simulink model "truck_fra_siden"  (R2023b)
settings: Solver=VariableStepAuto  StartTime=0.0  StopTime=100  MaxStep=0.01  RelTol=1e-3
values from neighbouring files (symbols this model uses):
  K_i = 10    [truck_fra_siden_script.m]
  K_p = 1400    [truck_fra_siden_script.m]
  v_r = 20    [truck_fra_siden_script.m]
settings Model: PacingRate=2  Creator=hansae  LastModifiedBy=fredr
settings SolverCC: AlgebraicLoopSolver=TrustRegion

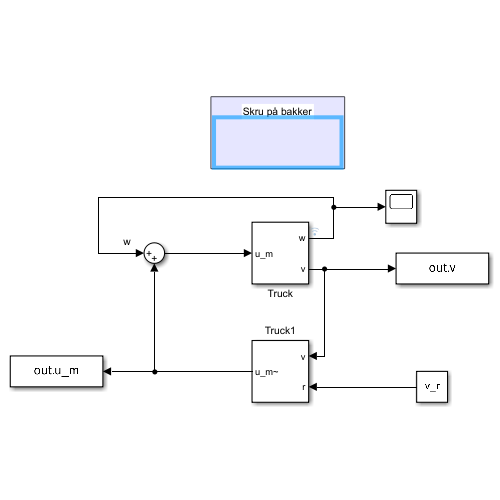
[thumbnail: Simulink's stored preview of the top-level diagram]
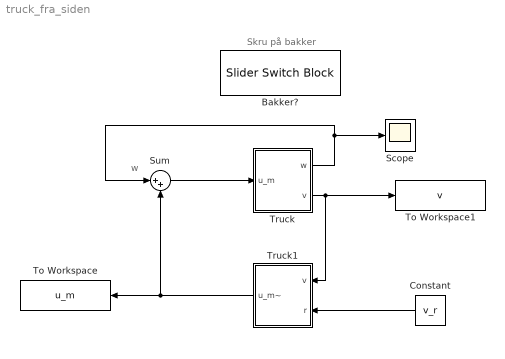
== system truck_fra_siden ==
  note: w
  note: Skru på bakker
  Bakker? : SliderSwitchBlock  LabelPosition=Hide
      settings: Values={{'Off', 'On'}, [0 1]}
  Constant : Constant  Value=v_r
  Scope : Scope
  Sum : Sum  Inputs=|++
  To Workspace : ToWorkspace  VariableName=u_m  SampleTime=-1
  To Workspace1 : ToWorkspace  VariableName=v  SampleTime=-1
  Truck : Subsystem
  Truck1 : Subsystem
  wires:
  Truck1/1(u_m~) -> Sum/2, To Workspace/1
  Truck/2(v) -> To Workspace1/1, Truck1/1(v)
  Constant/1 -> Truck1/2(r)
  Sum/1 -> Truck/1(u_m)
  Truck/1(w) -> Sum/1, Scope/1

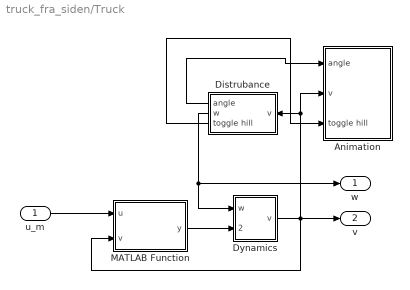
== system truck_fra_siden/Truck ==
  u_m : Inport
  Animation : Subsystem
  Distrubance : Subsystem
  Dynamics : Subsystem  ClipboardFcn=parameters_truck.m
  MATLAB Function : MATLAB Function  TreatAsAtomicUnit=on
  w : Outport
  v : Outport  Port=2
  wires:
  Dynamics/1(v) -> Animation/2(v), Distrubance/1(v), MATLAB Function/2(v), v/1
  Distrubance/1(angle) -> Animation/1(angle)
  u_m/1 -> MATLAB Function/1(u)
  MATLAB Function/1(y) -> Dynamics/2(u_m)
  Distrubance/2(w) -> w/1, Dynamics/1(w)
  Distrubance/3(toggle hill) -> Animation/3(toggle hill)

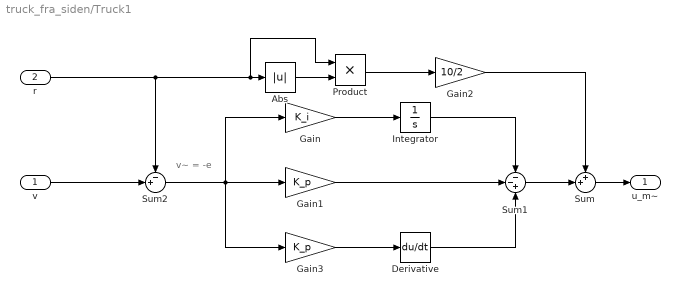
== system truck_fra_siden/Truck1 ==
  note: v~ = -e
  v : Inport
  r : Inport  Port=2
  Abs : Abs  SaturateOnIntegerOverflow=off
  Derivative : Derivative
  Gain : Gain  Gain=K_i
  Gain1 : Gain  Gain=K_p
  Gain2 : Gain  Gain=10/2
  Gain3 : Gain  Gain=K_p
  Integrator : Integrator
  Product : Product
  Sum : Sum  Inputs=++|
  Sum1 : Sum  Inputs=--+
  Sum2 : Sum  Inputs=-+|
  u_m~ : Outport
  wires:
  Sum/1 -> u_m~/1
  Gain/1 -> Integrator/1
  Sum1/1 -> Sum/2
  Gain1/1 -> Sum1/2
  Integrator/1 -> Sum1/1
  r/1 -> Product/1, Abs/1, Sum2/1
  Abs/1 -> Product/2
  Product/1 -> Gain2/1
  Gain2/1 -> Sum/1
  v/1 -> Sum2/2
  Sum2/1 -> Gain3/1, Gain1/1, Gain/1
  Gain3/1 -> Derivative/1
  Derivative/1 -> Sum1/3

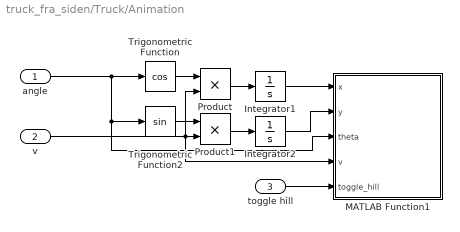
== system truck_fra_siden/Truck/Animation ==
  angle : Inport
  v : Inport  Port=2
  toggle hill : Inport  Port=3
  Integrator1 : Integrator
  Integrator2 : Integrator
  MATLAB Function1 : MATLAB Function  TreatAsAtomicUnit=on  SystemSampleTime=1/30
  Product : Product
  Product1 : Product
  Trigonometric Function : Trigonometry  Operator=cos
  Trigonometric Function2 : Trigonometry
  wires:
  Product/1 -> Integrator1/1
  Integrator1/1 -> MATLAB Function1/1(x)
  angle/1 -> Trigonometric Function2/1, MATLAB Function1/3(theta), Trigonometric Function/1
  v/1 -> MATLAB Function1/4(v), Product1/2, Product/2
  Integrator2/1 -> MATLAB Function1/2(y)
  Trigonometric Function/1 -> Product/1
  Product1/1 -> Integrator2/1
  Trigonometric Function2/1 -> Product1/1
  toggle hill/1 -> MATLAB Function1/5(toggle_hill)

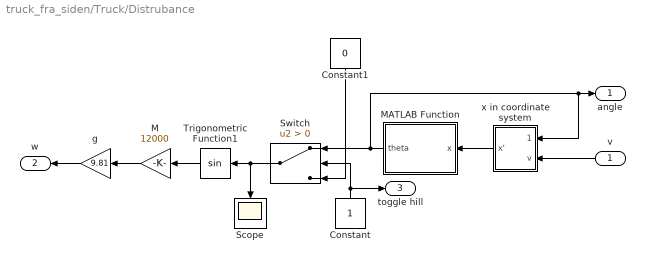
== system truck_fra_siden/Truck/Distrubance ==
  v : Inport
  Constant : Constant
  Constant1 : Constant  Value=0
  M : Gain  Gain=12000
  MATLAB Function : MATLAB Function  TreatAsAtomicUnit=on
  Scope : Scope
  Switch : Switch  Criteria=u2 > Threshold  SaturateOnIntegerOverflow=off  InputSameDT=off
  Trigonometric Function1 : Trigonometry
  g : Gain  Gain=9.81
  x in coordinate system : Subsystem
  angle : Outport
  w : Outport  Port=2
  toggle hill : Outport  Port=3
  wires:
  Trigonometric Function1/1 -> M/1
  M/1 -> g/1
  x in coordinate system/1(x') -> MATLAB Function/1(x)
  g/1 -> w/1
  v/1 -> x in coordinate system/2(v)
  Constant/1 -> Switch/2, toggle hill/1
  Switch/1 -> Trigonometric Function1/1, Scope/1
  MATLAB Function/1(theta) -> Switch/1, angle/1, x in coordinate system/1(theta)
  Constant1/1 -> Switch/3

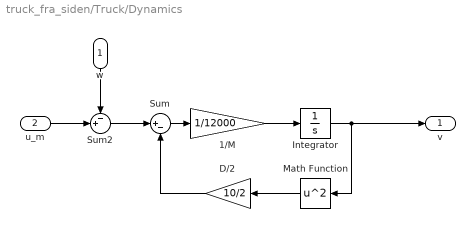
== system truck_fra_siden/Truck/Dynamics ==
  w : Inport
  u_m : Inport  Port=2
  1/M : Gain  Gain=1/12000
  D/2 : Gain  Gain=10/2
  Integrator : Integrator
  Math Function : Math  Operator=square
  Sum : Sum  Inputs=|+-
  Sum2 : Sum  Inputs=-+|
  v : Outport
  wires:
  Integrator/1 -> v/1, Math Function/1
  Sum/1 -> 1/M/1
  Sum2/1 -> Sum/1
  1/M/1 -> Integrator/1
  D/2/1 -> Sum/2
  Math Function/1 -> D/2/1
  w/1 -> Sum2/1
  u_m/1 -> Sum2/2

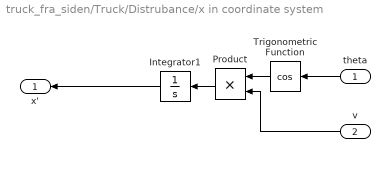
== system truck_fra_siden/Truck/Distrubance/x in coordinate system ==
  theta : Inport
  v : Inport  Port=2
  Integrator1 : Integrator
  Product : Product
  Trigonometric Function : Trigonometry  Operator=cos
  x' : Outport
  wires:
  Trigonometric Function/1 -> Product/1
  Product/1 -> Integrator1/1
  theta/1 -> Trigonometric Function/1
  Integrator1/1 -> x'/1
  v/1 -> Product/2

== matlab function truck_fra_siden/Truck/MATLAB Function ==
  data: u input; y output; v input
function y = saturation(u,v)
    Pmax = 400000;
    epsilon = 0.001;
    
    sat = Pmax/sqrt(v^2+epsilon);
    y = max(min(u,sat),-sat);

== matlab function truck_fra_siden/Truck/Distrubance/MATLAB Function ==
  data: theta output; x input
function theta = truck_road(x)
    %    height = 5;
    %    offset = 5;
    %    slope = 0.05;
    
    %    y = height*(tanh(slope*x-offset)+1);
    %    dy = height*slope*sech(offset-slope*x).^2;

    a = 5;
    b = 0.04;
    c = -0.2;
    d = 0.06;

    y = a*exp(sin(b*x))+c*exp(cos(d*x))-a*exp(sin(b*0))-c*exp(cos(d*0));
    dy = a*b*exp(sin(b*x)).*cos(b*x)-c*d*sin(d*x).*exp(cos(d*x));

    theta = atan2(dy,1);
end

== matlab function truck_fra_siden/Truck/Animation/MATLAB Function1 ==
  settings: updateMethod=DISCRETE
  data: x input; y input; theta input; v input; toggle_hill input
function plot_truck(x,y,theta,v,toggle_hill)
    % Parameters
    l = 8;
    persistent Truck;

    % Plotting Truck
    if isempty(Truck)
        Truck = initialize_plot();
    else
        if toggle_hill > 0.5
            update_truck_position(Truck,x,y,theta,v);
        else
            update_truck_position(Truck,x,0,0,v);
        end
    end    

    drawnow;

    % Functions
    function Truck = initialize_plot()
        % Initialize drawing time
        t_prev = 0;

        % Create figure
        figure('position',[100,100,1500,500]);
        clf; grid on; hold on; daspect([1,1,1]);
        xlim([-20, 50])
        ylim([-10, 10])
    
        % Initialize transformation objects
        Truck       = hgtransform('parent',gca);
        Wheel_back  = hgtransform('parent',Truck);
        Wheel_front = hgtransform('parent',Truck);
        
        % Chassie
        X = [0,0,l,l,7*l/8,2*l/3,2*l/3,0,0,11*l/18,11*l/18];
        Y = [l/10,0,0,l/6,l/3,l/3,l/10,l/10,2*l/5,2*l/5,l/10]+l/16;
        plot(X,Y,'parent',Truck,'color','k','linewidth',2);
        
        % Wheel back
        rectangle('Position',[l/8,0,l/8,l/8],'Curvature',1,'parent',Wheel_back,'edgecolor','k','linewidth',2)
        plot([l/8,2*l/8],[l/16,l/16],'parent',Wheel_back,'color','k','linewidth',2)
        plot([3*l/16,3*l/16],[0,l/8],'parent',Wheel_back,'color','k','linewidth',2)
        
        % Wheel front
        rectangle('Position',[6*l/8,0,l/8,l/8],'Curvature',1,'parent',Wheel_front,'edgecolor','k','linewidth',2)
        plot([6*l/8,7*l/8],[l/16,l/16],'parent',Wheel_front,'color','k','linewidth',2)
        plot([13*l/16,13*l/16],[0,l/8],'parent',Wheel_front,'color','k','linewidth',2)
    
        % Speedometer
        text(l/9,2*l/7,0,sprintf('%.2f m/s', 0),'parent',Truck)

        % Road trace
        x_road = linspace(min([-20, 50] + x)-100,max([-20, 50] + x)+1000,1000);
        if toggle_hill < 0.5
            y_road = 0*x_road;
        else
            [y_road,~] = truck_road(x_road);
        end

        plot(x_road,y_road, 'color', [0.5,0.5,0.5], 'linewidth', 3);
    end
    
    function update_truck_position(Truck,x,y,theta,dx)
        wheel_rotation = -16*x/l;

        if ishandle(Truck)
            set(Truck, 'Matrix', makehgtform('translate', [x, y, 0], 'zrotate', theta, 'translate', [-3*l/16, 0, 0]));
            
            children = get(Truck, 'Children');
            set(children(3), 'Matrix', makehgtform('translate', [13*l/16, l/16, 0], 'zrotate', wheel_rotation, 'translate', [-13*l/16, -l/16, 0]));
            set(children(4), 'Matrix', makehgtform('translate', [3*l/16, l/16, 0], 'zrotate', wheel_rotation, 'translate', [-3*l/16, -l/16, 0]));
    
            set(children(1), 'String', sprintf('%.2f m/s', dx));        
            set(children(1), 'Rotation', rad2deg(theta));
    
            xlim([-20, 50] + x)
            ylim([-10, 10] + y)
        end
    end

    function [y, theta] = truck_road(x)
        %    height = 5;
        %    offset = 5;
        %    slope = 0.05;
        
        %    y = height*(tanh(slope*x-offset)+1);
        %    dy = height*slope*sech(offset-slope*x).^2;
    
        a = 5;
        b = 0.04;
        c = -0.2;
        d = 0.06;
    
        y = a*exp(sin(b*x))+c*exp(cos(d*x))-a*exp(sin(b*0))-c*exp(cos(d*0));
        dy = a*b*exp(sin(b*x)).*cos(b*x)-c*d*sin(d*x).*exp(cos(d*x));
    
        theta = atan2(dy,1);
    end
end
